simulink model "modelstruktur"  (Simulink 7.8)
settings: Solver=ode45  StartTime=0.0  StopTime=10.0  RelTol=1e-3
settings Model: Creator=tina  LastModifiedBy=tina

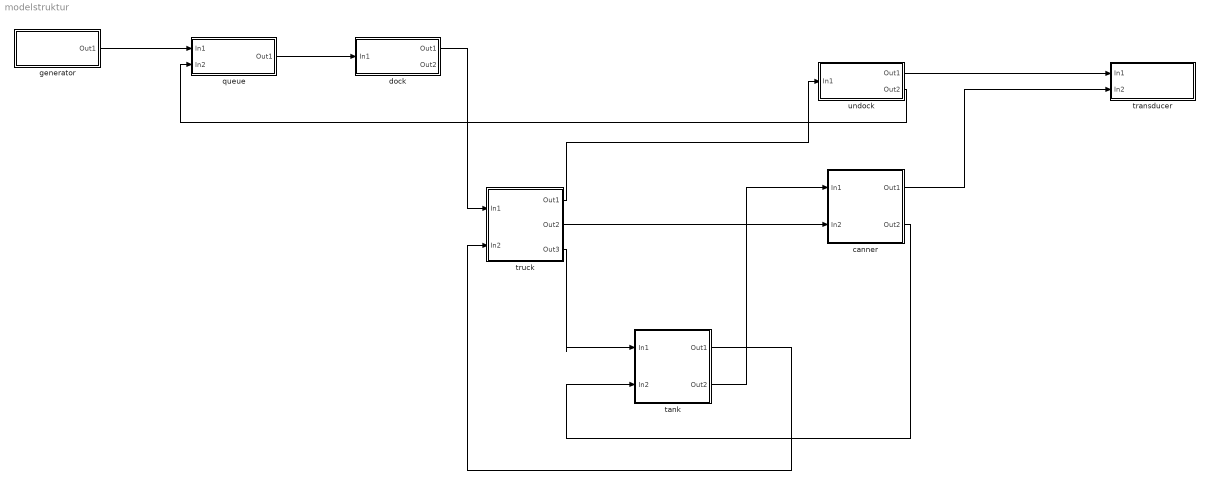
== system modelstruktur ==
  canner : Subsystem
  dock : Subsystem
  generator : Subsystem
  queue : Subsystem
  tank : Subsystem
  transducer : Subsystem
  truck : Subsystem
  undock : Subsystem
  wires:
  truck/1(Out1) -> undock/1(In1)
  canner/1(Out1) -> transducer/2(In2)
  queue/1(Out1) -> dock/1(In1)
  dock/1(Out1) -> truck/1(In1)
  tank/1(Out1) -> truck/2(In2)
  tank/2(Out2) -> canner/1(In1)
  truck/3(Out3) -> tank/1(In1)
  canner/2(Out2) -> tank/2(In2)
  truck/2(Out2) -> canner/2(In2)
  undock/1(Out1) -> transducer/1(In1)
  generator/1(Out1) -> queue/1(In1)
  undock/2(Out2) -> queue/2(In2)

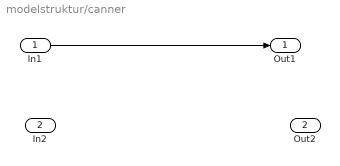
== system modelstruktur/canner ==
  In1 : Inport
  In2 : Inport  Port=2
  Out1 : Outport
  Out2 : Outport  Port=2
  wires:
  In1/1 -> Out1/1

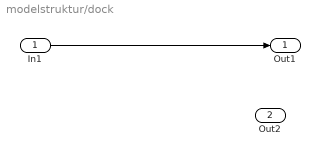
== system modelstruktur/dock ==
  In1 : Inport
  Out1 : Outport
  Out2 : Outport  Port=2
  wires:
  In1/1 -> Out1/1

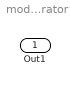
== system modelstruktur/generator ==
  Out1 : Outport
  wires:
  ? -> Out1/1

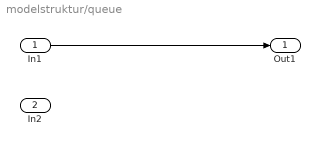
== system modelstruktur/queue ==
  In1 : Inport
  In2 : Inport  Port=2
  Out1 : Outport
  wires:
  In1/1 -> Out1/1

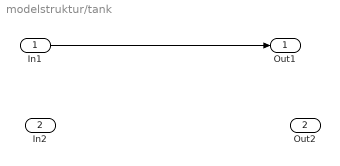
== system modelstruktur/tank ==
  In1 : Inport
  In2 : Inport  Port=2
  Out1 : Outport
  Out2 : Outport  Port=2
  wires:
  In1/1 -> Out1/1

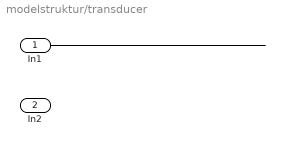
== system modelstruktur/transducer ==
  In1 : Inport
  In2 : Inport  Port=2
  wires:
  In1/1 -> ?

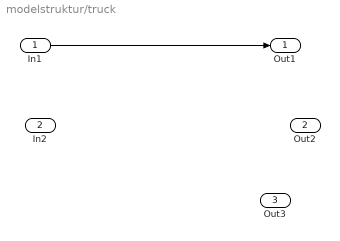
== system modelstruktur/truck ==
  In1 : Inport
  In2 : Inport  Port=2
  Out1 : Outport
  Out2 : Outport  Port=2
  Out3 : Outport  Port=3
  wires:
  In1/1 -> Out1/1

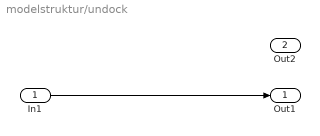
== system modelstruktur/undock ==
  In1 : Inport
  Out1 : Outport
  Out2 : Outport  Port=2
  wires:
  In1/1 -> Out1/1
